simulink model "testpendulum"  (R2017b)
settings: Solver=VariableStepAuto  StartTime=0.0  StopTime=10.0  MaxStep=0.01  RelTol=1e-3
undefined symbols (not defined in the file): g, l
settings Model: Creator=Zander  LastModifiedBy=Zander

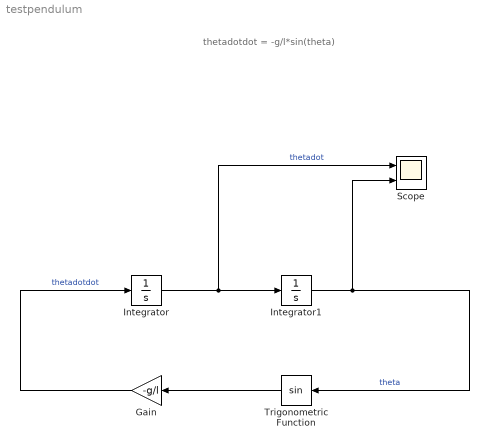
== system testpendulum ==
  note: thetadotdot = -g/l*sin(theta)
  Gain : Gain  Gain=-g/l
  Integrator : Integrator
  Integrator1 : Integrator  InitialCondition=40
  Scope : Scope  NumInputPorts=2
  Trigonometric Function : Trigonometry
  wires:
  Gain/1 -> Integrator/1  "thetadotdot"
  Integrator/1 -> Scope/1, Integrator1/1  "thetadot"
  Integrator1/1 -> Scope/2, Trigonometric Function/1  "theta"
  Trigonometric Function/1 -> Gain/1
